simulink model "modelo_b"  (R2026a)
settings: Solver=ode4  StopTime=t_final  FixedStep=dt
values from neighbouring files (symbols this model uses):
  theta = 5    [init.m]
settings Model: Creator=honda  LastModifiedBy=honda

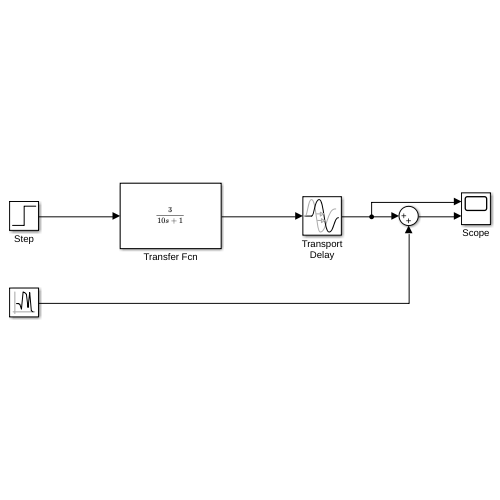
[thumbnail: Simulink's stored preview of the top-level diagram]
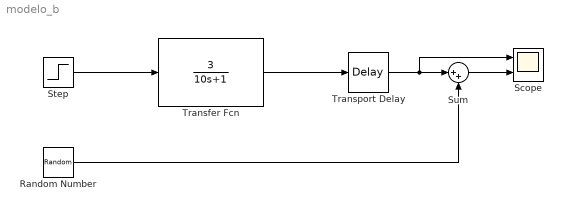
== system modelo_b ==
  Random Number : RandomNumber  Variance=1e-6  SampleTime=0.01
  Scope : Scope  NumInputPorts=2
      settings: ActiveDisplayYMinimum=-0.0324329981496793  ActiveDisplayYMaximum=0.26316947065042862  DataLoggingVariableName=dados_b
  Step : Step  Time=0  FinalValue=u0  SampleTime=0
  Sum : Sum  Inputs=|++
  Transfer Fcn : TransferFcn  Numerator=[3]  Denominator=[10 1]
  Transport Delay : TransportDelay  DelayTime=theta
  wires:
  Step/1 -> Transfer Fcn/1
  Transfer Fcn/1 -> Transport Delay/1
  Transport Delay/1 -> Scope/1, Sum/1
  Sum/1 -> Scope/2
  Random Number/1 -> Sum/2
